simulink model "Fig49"  (R2014b)
settings: Solver=ode45  StartTime=0.0  StopTime=.005  RelTol=1e-3
libraries: dspquant2 x2, dspsigops x1, dsparch4 x1
settings Model: Creator=Dennis Silage  LastModifiedBy=Silage
settings DataIOCC: SignalLoggingSaveFormat=ModelDataLogs
settings OptimizationCC: ExpressionDepthLimit=2147483647  InitFltsAndDblsToZero=on
settings DebuggingCC: UnderspecifiedInitializationDetection=Classic  MergeDetectMultiDrivingBlocksExec=none  FcnCallInpInsideContextMsg=UseLocalSettings  StateNameClashWarn=warning
settings GRTTargetCC: CombineOutputUpdateFcns=off  GRTInterface=on

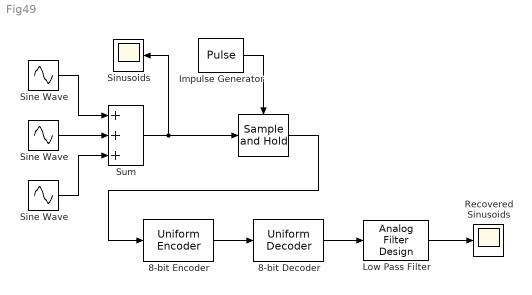
== system Fig49 ==
  "   " : dspsigops/Sample and Hold  trig=Rising edge  initCond=0  latchinput=off
  " Sine Wave " : Sin  Amplitude=0.2  Frequency=5000*pi  SampleTime=1.25e-6
  8-bit Decoder : dspquant2/Uniform Decoder  peak=1.28  bits=8  overflowMode=Saturate  otype=Double
  8-bit Encoder : dspquant2/Uniform Encoder  peak=1.28  bits=8  otype=Signed integer
  Impulse Generator : DiscretePulseGenerator  Period=100  SampleTime=1.25e-6
  Low Pass Filter : dsparch4/Analog Filter Design  method=Butterworth  filttype=Lowpass  N=9  Wlo=6000*pi  Whi=80  Rp=2  Rs=40
  Recovered Sinusoids : Scope
      settings: YMin=-1.5  YMax=1.5  SaveName=ScopeData4
  Sine Wave : Sin  Frequency=1000*pi  SampleTime=1.25e-6
  "Sine Wave " : Sin  Amplitude=0.5  Frequency=3000*pi  SampleTime=1.25e-6
  Sinusoids : Scope
      settings: YMin=-1.5  YMax=1.5
  Sum : Sum  Inputs=+++
  wires:
  "Sine Wave "/1 -> Sum/2
  " Sine Wave "/1 -> Sum/3
  Sine Wave/1 -> Sum/1
  Sum/1 -> "   "/1, Sinusoids/1
  Impulse Generator/1 -> "   "/Trigger
  "   "/1 -> 8-bit Encoder/1
  8-bit Encoder/1 -> 8-bit Decoder/1
  8-bit Decoder/1 -> Low Pass Filter/1
  Low Pass Filter/1 -> Recovered Sinusoids/1
